simulink model "slab03"  (R2023b)
settings: Solver=VariableStepAuto  StartTime=0.0  StopTime=10.0  RelTol=1e-3
values from neighbouring files (symbols this model uses):
  C = [1 0 0]    [lab3.m]
undefined symbols (not defined in the file or in its folder): fg_chua, ga, mu_chua, ref_chua, u_chua
settings Model: Creator=s331564  LastModifiedBy=luigi

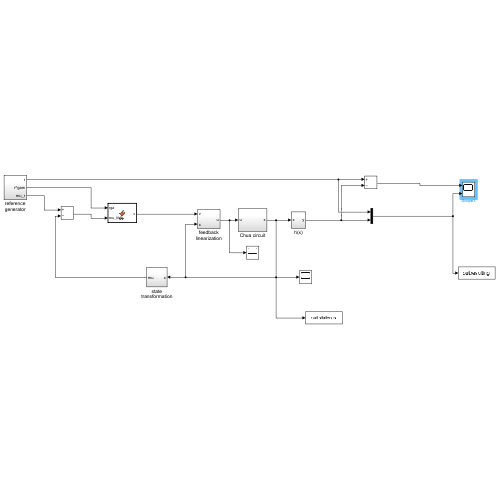
[thumbnail: Simulink's stored preview of the top-level diagram]
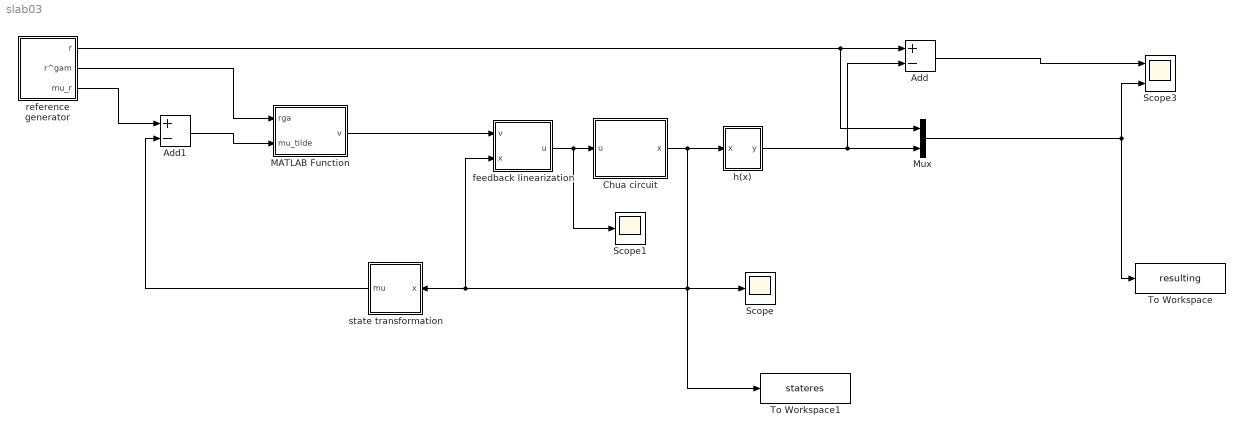
== system slab03 ==
  Add : Sum  Inputs=+-
  Add1 : Sum  Inputs=+-
  Chua circuit : Subsystem
  MATLAB Function : MATLAB Function  TreatAsAtomicUnit=on
  Mux : Mux  Inputs=2
  Scope : Scope
  Scope1 : Scope
  Scope3 : Scope  NumInputPorts=2
  To Workspace : ToWorkspace  VariableName=resulting  SaveFormat=Timeseries  SampleTime=-1
  To Workspace1 : ToWorkspace  VariableName=stateres  SaveFormat=Timeseries  SampleTime=-1
  feedback linearization : Subsystem
  h(x) : Subsystem
  reference generator : Subsystem
  state transformation : Subsystem
  wires:
  feedback linearization/1(u) -> Scope1/1, Chua circuit/1(u)
  Chua circuit/1(x) -> h(x)/1(x), To Workspace1/1, feedback linearization/2(x), state transformation/1(x), Scope/1
  h(x)/1(y) -> Add/2, Mux/2
  Mux/1 -> Scope3/2, To Workspace/1
  reference generator/1(r) -> Mux/1, Add/1
  Add/1 -> Scope3/1
  state transformation/1(mu) -> Add1/2
  reference generator/3(mu_r) -> Add1/1
  reference generator/2(r^gam) -> MATLAB Function/1(rga)
  MATLAB Function/1(v) -> feedback linearization/1(v)
  Add1/1 -> MATLAB Function/2(mu_tilde)

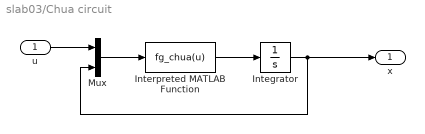
== system slab03/Chua circuit ==
  u : Inport
  Integrator : Integrator  InitialCondition=[0; 0; 0]
  Interpreted MATLAB Function : MATLABFcn  MATLABFcn=fg_chua(u)
  Mux : Mux  Inputs=2
  x : Outport  VectorParamsAs1DForOutWhenUnconnected=off
  wires:
  u/1 -> Mux/1
  Interpreted MATLAB Function/1 -> Integrator/1
  Integrator/1 -> Mux/2, x/1
  Mux/1 -> Interpreted MATLAB Function/1

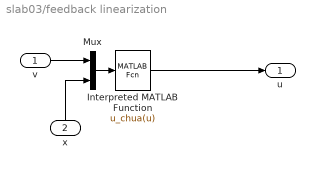
== system slab03/feedback linearization ==
  v : Inport
  x : Inport  Port=2
  Interpreted MATLAB Function : MATLABFcn  MATLABFcn=u_chua(u)  OutputSignalType=real
  Mux : Mux  Inputs=2
  u : Outport  VectorParamsAs1DForOutWhenUnconnected=off
  wires:
  x/1 -> Mux/2
  Mux/1 -> Interpreted MATLAB Function/1
  v/1 -> Mux/1
  Interpreted MATLAB Function/1 -> u/1

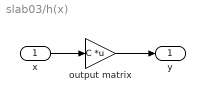
== system slab03/h(x) ==
  x : Inport
  output matrix : Gain  Gain=C  Multiplication=Matrix(K*u)
  y : Outport  VectorParamsAs1DForOutWhenUnconnected=off
  wires:
  x/1 -> output matrix/1
  output matrix/1 -> y/1

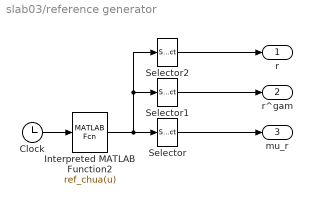
== system slab03/reference generator ==
  Clock : Clock
  Interpreted MATLAB Function2 : MATLABFcn  MATLABFcn=ref_chua(u)
  Selector : Selector  InputPortWidth=ga+1  IndexOptions=Index vector (dialog)  Indices=1:ga  OutputSizes=1
  Selector1 : Selector  InputPortWidth=ga+1  IndexOptions=Index vector (dialog)  Indices=ga+1  OutputSizes=1
  Selector2 : Selector  InputPortWidth=ga+1  IndexOptions=Index vector (dialog)  Indices=1  OutputSizes=1
  r : Outport  VectorParamsAs1DForOutWhenUnconnected=off
  r^gam : Outport  Port=2  VectorParamsAs1DForOutWhenUnconnected=off
  mu_r : Outport  Port=3  VectorParamsAs1DForOutWhenUnconnected=off
  wires:
  Clock/1 -> Interpreted MATLAB Function2/1
  Selector1/1 -> r^gam/1
  Selector2/1 -> r/1
  Interpreted MATLAB Function2/1 -> Selector2/1, Selector1/1, Selector/1
  Selector/1 -> mu_r/1

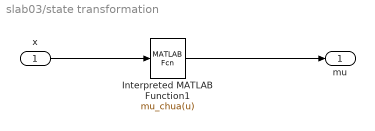
== system slab03/state transformation ==
  x : Inport
  Interpreted MATLAB Function1 : MATLABFcn  MATLABFcn=mu_chua(u)
  mu : Outport  VectorParamsAs1DForOutWhenUnconnected=off
  wires:
  x/1 -> Interpreted MATLAB Function1/1
  Interpreted MATLAB Function1/1 -> mu/1

== matlab function slab03/MATLAB Function ==
  data: rga input; v output; mu_tilde input
function v = fcn(rga, mu_tilde)

k2 = 30;
k1 =50;
eta = 5;
s = mu_tilde(2) + k2 * mu_tilde(1);

v = rga+ k2*mu_tilde(2)+k1*sign(eta*s);
end
